simulink model "PID_PFL_3D_winds"  (R2022b)
settings: Solver=ode15s  StartTime=0.0  StopTime=0.8803  RelTol=1e-3
values from neighbouring files (symbols this model uses):
  theta1x_in = pinput(4 : 3 + n)    [Animation_3D.m]    (also in Constraint_3D_WCW.m = pinput(4 : 3+n); Cost_3D_WCW.m = pinput(4 : 3+n))
  theta1y_in = pinput(4 + n : 3 + 2*n)    [Animation_3D.m]    (also in Constraint_3D_WCW.m = pinput(4+n : 3+2*n); Cost_3D_WCW.m = pinput(4+n : 3+2*n))
  theta2_in = pinput(4 + 2*n : 3 + 3*n)    [Animation_3D.m]    (also in Constraint_3D_WCW.m = pinput(4+2*n : 3+3*n); Cost_3D_WCW.m = pinput(4+2*n : 3+3*n))
  timeVec = linspace(0, simTime, n)'    [Animation_3D.m]    (also in Main_3D_WCW.m = linspace(0, xmin(1), n)')
undefined symbols (not defined in the file or in its folder): sigbuilder_block, windSpeed
libraries: nesl_utility x6, sm_lib x4, slpidlib x3, simulink_extras x1
(part 1 of 2)
settings Model: Creator=Lenovo  LastModifiedBy=Stanley Mbewe
settings OptimizationCC: ReuseModelBlockBuffer=on

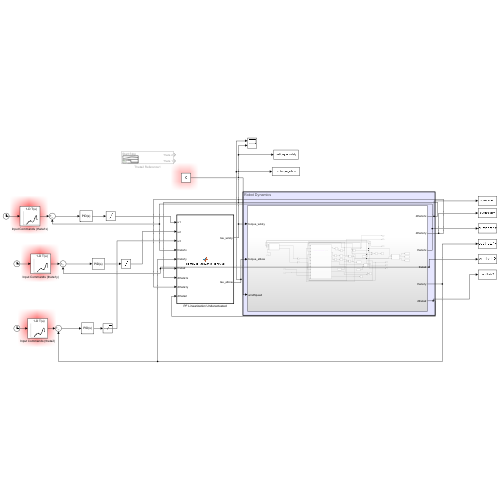
[thumbnail: Simulink's stored preview of the top-level diagram]
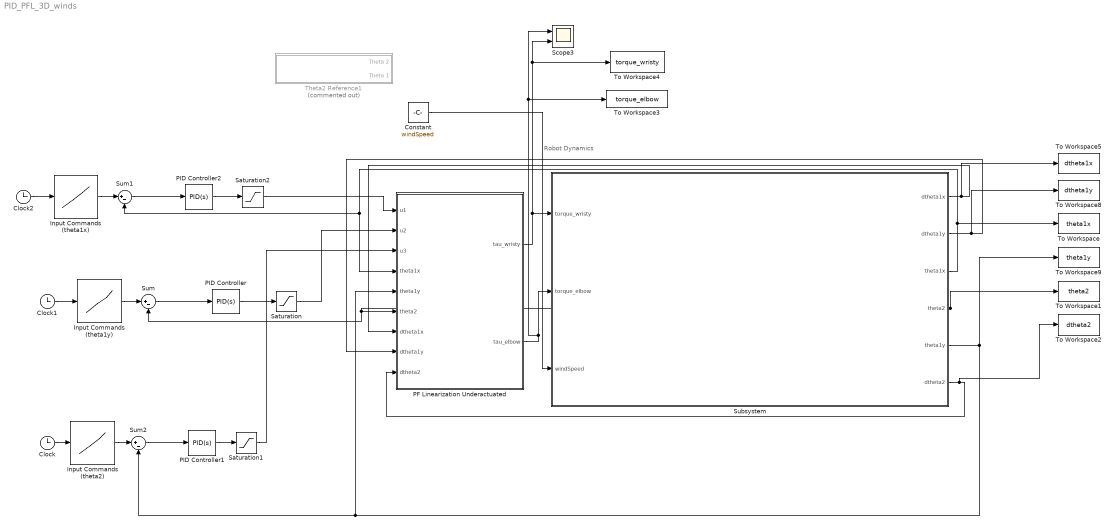
== system PID_PFL_3D_winds ==
  note: Robot Dynamics
  Clock : Clock
  Clock1 : Clock
  Clock2 : Clock
  Constant : Constant  Value=windSpeed
  Input Commands (theta1x) : Lookup_n-D  NumberOfTableDimensions=1  BreakpointsForDimension1=timeVec  Table=theta1x_in  InterpMethod=Cubic spline  InternalRulePriority=Speed  RndMeth=Simplest
  Input Commands (theta1y) : Lookup_n-D  NumberOfTableDimensions=1  BreakpointsForDimension1=timeVec  Table=theta1y_in  InterpMethod=Cubic spline  InternalRulePriority=Speed  RndMeth=Simplest
  Input Commands (theta2) : Lookup_n-D  NumberOfTableDimensions=1  LookupTableObject=theta1_in  BreakpointsForDimension1=timeVec  Table=theta2_in  InterpMethod=Cubic spline  InternalRulePriority=Speed  RndMeth=Simplest
  PF Linearization Underactuated : MATLAB Function  TreatAsAtomicUnit=on
  PID Controller : slpidlib/PID Controller  Controller=PID  Form=Parallel  TimeDomain=Continuous-time  UseExternalTs=off  SampleTime=-1  IntegratorMethod=Forward Euler  FilterMethod=Forward Euler  ControllerParametersSource=internal  P=149  I=10.1896438485082  UseKiTs=off  D=114  N=100  UseFilter=on  TunerSelectOption=Transfer Function Based (PID Tuner App)  InitialConditionSource=internal  InitialConditionForIntegrator=0  InitialConditionForFilter=0  DifferentiatorICPrevScaledInput=0  ExternalReset=none  TrackingMode=off  Kt=1  LimitOutput=off  SatLimitsSource=internal  UpperSaturationLimit=inf  LowerSaturationLimit=-inf  LinearizeAsGain=on  AntiWindupMode=none  Kb=1  LimitIntegrator=off  UpperIntegratorSaturationLimit=inf  LowerIntegratorSaturationLimit=-inf  POutMin=[]  POutMax=[]  IOutMin=[]  IOutMax=[]  DOutMin=[]  DOutMax=[]  NOutMin=[]  NOutMax=[]  SumOutMin=[]  SumOutMax=[]  SaturationOutMin=[]  SaturationOutMax=[]  PParamMin=[]  PParamMax=[]  IParamMin=[]  IParamMax=[]  DParamMin=[]  DParamMax=[]  NParamMin=[]  NParamMax=[]  KbParamMin=[]  KbParamMax=[]  KtParamMin=[]  KtParamMax=[]  KbOutMin=[]  KbOutMax=[]  KtOutMin=[]  KtOutMax=[]  IntegratorOutMin=[]  IntegratorOutMax=[]  FilterOutMin=[]  FilterOutMax=[]  SumI1OutMin=[]  SumI1OutMax=[]  SumI2OutMin=[]  SumI2OutMax=[]  SumI3OutMin=[]  SumI3OutMax=[]  SumI4OutMin=[]  SumI4OutMax=[]  SumDOutMin=[]  SumDOutMax=[]  DifferentiatorOutMin=[]  DifferentiatorOutMax=[]  FilterDiffOutCoefMin=[]  FilterDiffOutCoefMax=[]  ReciprocalOutMin=[]  ReciprocalOutMax=[]  SumDenOutMin=[]  SumDenOutMax=[]  SumNumOutMin=[]  SumNumOutMax=[]  DivideOutMin=[]  DivideOutMax=[]  UdiffTsProdOutMin=[]  UdiffTsProdOutMax=[]  NTsProdOutMin=[]  NTsProdOutMax=[]  UintegralTsProdOutMin=[]  UintegralTsProdOutMax=[]  UngainTsProdOutMin=[]  UngainTsProdOutMax=[]  ClampingZeroOutDataTypeStr=Inherit: Inherit via back propagation  ClampingZeroOutMin=[]  ClampingZeroOutMax=[]  FilterDenConstantOutDataTypeStr=Inherit: Inherit via back propagation  FilterDenConstantOutMin=[]  FilterDenConstantOutMax=[]  PCopyOutDataTypeStr=Inherit: Inherit via back propagation  PCopyOutMin=[]  PCopyOutMax=[]  NCopyOutDataTypeStr=Inherit: Inherit via back propagation  NCopyOutMin=[]  NCopyOutMax=[]  IntegratorContinuousStateAttributes=''  IntegratorStateMustResolveToSignalObject=off  IntegratorRTWStateStorageClass=Auto  FilterContinuousStateAttributes=''  FilterStateMustResolveToSignalObject=off  FilterRTWStateStorageClass=Auto  ParallelPVariant=InternalParameters  IdealPVariant=Disabled  IVariant=InternalParameters  DVariant=InternalParameters  IntegratorVariant=Continuous  SatVariant=Disabled  AWVariant=Passthrough  PCopyVariant=Disabled  TRVariant=Disabled  FdbkBlocksVariant=Forward  IdealPFdbkVariant=Disabled  SatFdbkVariant=Disabled  DerivativeFilterVariant=ContFilter  NVariant=InternalParameters  NCopyVariant=Disabled  FilterICVariant=InternalICsFilter  IntegratorICVariant=InternalICs  ExternalResetVariant=Disabled  TRSumVariant=Passthrough  SumFdbkVariant=Disabled  SumVariant=Sum_PID  TsampFilterVariant=InternalTs  TsampNgainVariant=Passthrough  TsampIntegralVariant=Passthrough  ExternalSaturationOutDataTypeStr=Inherit: Same as second input
  PID Controller1 : slpidlib/PID Controller  Controller=PID  Form=Parallel  TimeDomain=Continuous-time  UseExternalTs=off  SampleTime=-1  IntegratorMethod=Forward Euler  FilterMethod=Forward Euler  ControllerParametersSource=internal  P=149  I=10.1896438485082  UseKiTs=off  D=114  N=100  UseFilter=on  TunerSelectOption=Transfer Function Based (PID Tuner App)  InitialConditionSource=internal  InitialConditionForIntegrator=0  InitialConditionForFilter=0  DifferentiatorICPrevScaledInput=0  ExternalReset=none  TrackingMode=off  Kt=1  LimitOutput=off  SatLimitsSource=internal  UpperSaturationLimit=inf  LowerSaturationLimit=-inf  LinearizeAsGain=on  AntiWindupMode=none  Kb=1  LimitIntegrator=off  UpperIntegratorSaturationLimit=inf  LowerIntegratorSaturationLimit=-inf  POutMin=[]  POutMax=[]  IOutMin=[]  IOutMax=[]  DOutMin=[]  DOutMax=[]  NOutMin=[]  NOutMax=[]  SumOutMin=[]  SumOutMax=[]  SaturationOutMin=[]  SaturationOutMax=[]  PParamMin=[]  PParamMax=[]  IParamMin=[]  IParamMax=[]  DParamMin=[]  DParamMax=[]  NParamMin=[]  NParamMax=[]  KbParamMin=[]  KbParamMax=[]  KtParamMin=[]  KtParamMax=[]  KbOutMin=[]  KbOutMax=[]  KtOutMin=[]  KtOutMax=[]  IntegratorOutMin=[]  IntegratorOutMax=[]  FilterOutMin=[]  FilterOutMax=[]  SumI1OutMin=[]  SumI1OutMax=[]  SumI2OutMin=[]  SumI2OutMax=[]  SumI3OutMin=[]  SumI3OutMax=[]  SumI4OutMin=[]  SumI4OutMax=[]  SumDOutMin=[]  SumDOutMax=[]  DifferentiatorOutMin=[]  DifferentiatorOutMax=[]  FilterDiffOutCoefMin=[]  FilterDiffOutCoefMax=[]  ReciprocalOutMin=[]  ReciprocalOutMax=[]  SumDenOutMin=[]  SumDenOutMax=[]  SumNumOutMin=[]  SumNumOutMax=[]  DivideOutMin=[]  DivideOutMax=[]  UdiffTsProdOutMin=[]  UdiffTsProdOutMax=[]  NTsProdOutMin=[]  NTsProdOutMax=[]  UintegralTsProdOutMin=[]  UintegralTsProdOutMax=[]  UngainTsProdOutMin=[]  UngainTsProdOutMax=[]  ClampingZeroOutDataTypeStr=Inherit: Inherit via back propagation  ClampingZeroOutMin=[]  ClampingZeroOutMax=[]  FilterDenConstantOutDataTypeStr=Inherit: Inherit via back propagation  FilterDenConstantOutMin=[]  FilterDenConstantOutMax=[]  PCopyOutDataTypeStr=Inherit: Inherit via back propagation  PCopyOutMin=[]  PCopyOutMax=[]  NCopyOutDataTypeStr=Inherit: Inherit via back propagation  NCopyOutMin=[]  NCopyOutMax=[]  IntegratorContinuousStateAttributes=''  IntegratorStateMustResolveToSignalObject=off  IntegratorRTWStateStorageClass=Auto  FilterContinuousStateAttributes=''  FilterStateMustResolveToSignalObject=off  FilterRTWStateStorageClass=Auto  ParallelPVariant=InternalParameters  IdealPVariant=Disabled  IVariant=InternalParameters  DVariant=InternalParameters  IntegratorVariant=Continuous  SatVariant=Disabled  AWVariant=Passthrough  PCopyVariant=Disabled  TRVariant=Disabled  FdbkBlocksVariant=Forward  IdealPFdbkVariant=Disabled  SatFdbkVariant=Disabled  DerivativeFilterVariant=ContFilter  NVariant=InternalParameters  NCopyVariant=Disabled  FilterICVariant=InternalICsFilter  IntegratorICVariant=InternalICs  ExternalResetVariant=Disabled  TRSumVariant=Passthrough  SumFdbkVariant=Disabled  SumVariant=Sum_PID  TsampFilterVariant=InternalTs  TsampNgainVariant=Passthrough  TsampIntegralVariant=Passthrough  ExternalSaturationOutDataTypeStr=Inherit: Same as second input
  PID Controller2 : slpidlib/PID Controller  Controller=PID  Form=Parallel  TimeDomain=Continuous-time  UseExternalTs=off  SampleTime=-1  IntegratorMethod=Forward Euler  FilterMethod=Forward Euler  ControllerParametersSource=internal  P=149  I=10.1896438485082  UseKiTs=off  D=114  N=100  UseFilter=on  TunerSelectOption=Transfer Function Based (PID Tuner App)  InitialConditionSource=internal  InitialConditionForIntegrator=0  InitialConditionForFilter=0  DifferentiatorICPrevScaledInput=0  ExternalReset=none  TrackingMode=off  Kt=1  LimitOutput=off  SatLimitsSource=internal  UpperSaturationLimit=inf  LowerSaturationLimit=-inf  LinearizeAsGain=on  AntiWindupMode=none  Kb=1  LimitIntegrator=off  UpperIntegratorSaturationLimit=inf  LowerIntegratorSaturationLimit=-inf  POutMin=[]  POutMax=[]  IOutMin=[]  IOutMax=[]  DOutMin=[]  DOutMax=[]  NOutMin=[]  NOutMax=[]  SumOutMin=[]  SumOutMax=[]  SaturationOutMin=[]  SaturationOutMax=[]  PParamMin=[]  PParamMax=[]  IParamMin=[]  IParamMax=[]  DParamMin=[]  DParamMax=[]  NParamMin=[]  NParamMax=[]  KbParamMin=[]  KbParamMax=[]  KtParamMin=[]  KtParamMax=[]  KbOutMin=[]  KbOutMax=[]  KtOutMin=[]  KtOutMax=[]  IntegratorOutMin=[]  IntegratorOutMax=[]  FilterOutMin=[]  FilterOutMax=[]  SumI1OutMin=[]  SumI1OutMax=[]  SumI2OutMin=[]  SumI2OutMax=[]  SumI3OutMin=[]  SumI3OutMax=[]  SumI4OutMin=[]  SumI4OutMax=[]  SumDOutMin=[]  SumDOutMax=[]  DifferentiatorOutMin=[]  DifferentiatorOutMax=[]  FilterDiffOutCoefMin=[]  FilterDiffOutCoefMax=[]  ReciprocalOutMin=[]  ReciprocalOutMax=[]  SumDenOutMin=[]  SumDenOutMax=[]  SumNumOutMin=[]  SumNumOutMax=[]  DivideOutMin=[]  DivideOutMax=[]  UdiffTsProdOutMin=[]  UdiffTsProdOutMax=[]  NTsProdOutMin=[]  NTsProdOutMax=[]  UintegralTsProdOutMin=[]  UintegralTsProdOutMax=[]  UngainTsProdOutMin=[]  UngainTsProdOutMax=[]  ClampingZeroOutDataTypeStr=Inherit: Inherit via back propagation  ClampingZeroOutMin=[]  ClampingZeroOutMax=[]  FilterDenConstantOutDataTypeStr=Inherit: Inherit via back propagation  FilterDenConstantOutMin=[]  FilterDenConstantOutMax=[]  PCopyOutDataTypeStr=Inherit: Inherit via back propagation  PCopyOutMin=[]  PCopyOutMax=[]  NCopyOutDataTypeStr=Inherit: Inherit via back propagation  NCopyOutMin=[]  NCopyOutMax=[]  IntegratorContinuousStateAttributes=''  IntegratorStateMustResolveToSignalObject=off  IntegratorRTWStateStorageClass=Auto  FilterContinuousStateAttributes=''  FilterStateMustResolveToSignalObject=off  FilterRTWStateStorageClass=Auto  ParallelPVariant=InternalParameters  IdealPVariant=Disabled  IVariant=InternalParameters  DVariant=InternalParameters  IntegratorVariant=Continuous  SatVariant=Disabled  AWVariant=Passthrough  PCopyVariant=Disabled  TRVariant=Disabled  FdbkBlocksVariant=Forward  IdealPFdbkVariant=Disabled  SatFdbkVariant=Disabled  DerivativeFilterVariant=ContFilter  NVariant=InternalParameters  NCopyVariant=Disabled  FilterICVariant=InternalICsFilter  IntegratorICVariant=InternalICs  ExternalResetVariant=Disabled  TRSumVariant=Passthrough  SumFdbkVariant=Disabled  SumVariant=Sum_PID  TsampFilterVariant=InternalTs  TsampNgainVariant=Passthrough  TsampIntegralVariant=Passthrough  ExternalSaturationOutDataTypeStr=Inherit: Same as second input
  Saturation : Saturate  UpperLimit=10  LowerLimit=-10
  Saturation1 : Saturate  UpperLimit=50  LowerLimit=-50
  Saturation2 : Saturate  UpperLimit=10  LowerLimit=-10
  Scope3 : Scope  NumInputPorts=2
  Subsystem : Subsystem
  Sum : Sum  Inputs=|+-
  Sum1 : Sum  Inputs=|+-
  Sum2 : Sum  Inputs=|+-
  Theta2 Reference1 : Subsystem  Tag=STV Subsys  Commented=on  LoadFcn=sigbuilder_block('load');  StartFcn=sigbuilder_block('start');  StopFcn=sigbuilder_block('stop');  ClipboardFcn=sigbuilder_block('clipboard');  mask(Sigbuilder block){tuvar=[0:10]}
      mask help: Sigbuilder GUI
      mask init:
      | if ~strcmp(get_param(bdroot(gcbh),'SimulationStatus'),'stopped') tuvar = sigbuilder_block('maskInit'); end
      settings: CopyFcn=sigbuilder_block('copy');  DeleteFcn=sigbuilder_block('delete');  ModelCloseFcn=sigbuilder_block('modelClose');  PreSaveFcn=sigbuilder_block('preSave');  PauseFcn=sigbuilder_block('pause')  ContinueFcn=sigbuilder_block('continue')  NameChangeFcn=sigbuilder_block('namechange');  OpenFcn=sigbuilder_block('open',[200.4 71.4 762 360.6 ]);  CloseFcn=sigbuilder_block('close');
      mask Display: plot(0, 0, 100, 100,[2, 2, 32, 32, 2], [68, 8, 8, 68, 68],[32, 2], [38, 38], [32, 19, 2],[53, 60, 44], [32, 17, 17, 2],[16, 16, 31, 31]);txt = getActiveGroup(gcbh);text(2, 100, txt,'verticalAlignment', 'top');
  To Workspace : ToWorkspace  VariableName=theta1x  SampleTime=0.01
  To Workspace1 : ToWorkspace  VariableName=theta2  SampleTime=0.01
  To Workspace2 : ToWorkspace  VariableName=dtheta2  SampleTime=0.01
  To Workspace3 : ToWorkspace  VariableName=torque_elbow  SampleTime=0.01
  To Workspace4 : ToWorkspace  VariableName=torque_wristy  SampleTime=0.01
  To Workspace5 : ToWorkspace  VariableName=dtheta1x  SampleTime=0.01
  To Workspace8 : ToWorkspace  VariableName=dtheta1y  SampleTime=0.01
  To Workspace9 : ToWorkspace  VariableName=theta1y  SampleTime=0.01
  wires:
  Sum/1 -> PID Controller/1
  Sum2/1 -> PID Controller1/1
  PID Controller/1 -> Saturation/1
  PID Controller1/1 -> Saturation1/1
  Clock/1 -> Input Commands (theta2)/1
  Clock1/1 -> Input Commands (theta1y)/1
  PF Linearization Underactuated/1(tau_wristy) -> To Workspace4/1, Scope3/2, Subsystem/1(torque_wristy)
  PF Linearization Underactuated/2(tau_elbow) -> Scope3/1, To Workspace3/1, Subsystem/2(torque_elbow)
  Subsystem/4(theta2) -> To Workspace1/1, PF Linearization Underactuated/6(theta2), Sum/2
  Subsystem/5(theta1y) -> PF Linearization Underactuated/5(theta1y), Sum2/2, To Workspace9/1
  Subsystem/3(theta1x) -> To Workspace/1, Sum1/2, PF Linearization Underactuated/4(theta1x)
  Subsystem/1(dtheta1x) -> To Workspace5/1, PF Linearization Underactuated/7(dtheta1x)
  Subsystem/2(dtheta1y) -> To Workspace8/1, PF Linearization Underactuated/8(dtheta1y)
  Subsystem/6(dtheta2) -> To Workspace2/1, PF Linearization Underactuated/9(dtheta2)
  Input Commands (theta2)/1 -> Sum2/1
  Input Commands (theta1y)/1 -> Sum/1
  Input Commands (theta1x)/1 -> Sum1/1
  Clock2/1 -> Input Commands (theta1x)/1
  PID Controller2/1 -> Saturation2/1
  Sum1/1 -> PID Controller2/1
  Saturation2/1 -> PF Linearization Underactuated/1(u1)
  Saturation/1 -> PF Linearization Underactuated/2(u2)
  Saturation1/1 -> PF Linearization Underactuated/3(u3)
  Constant/1 -> Subsystem/3(windSpeed)

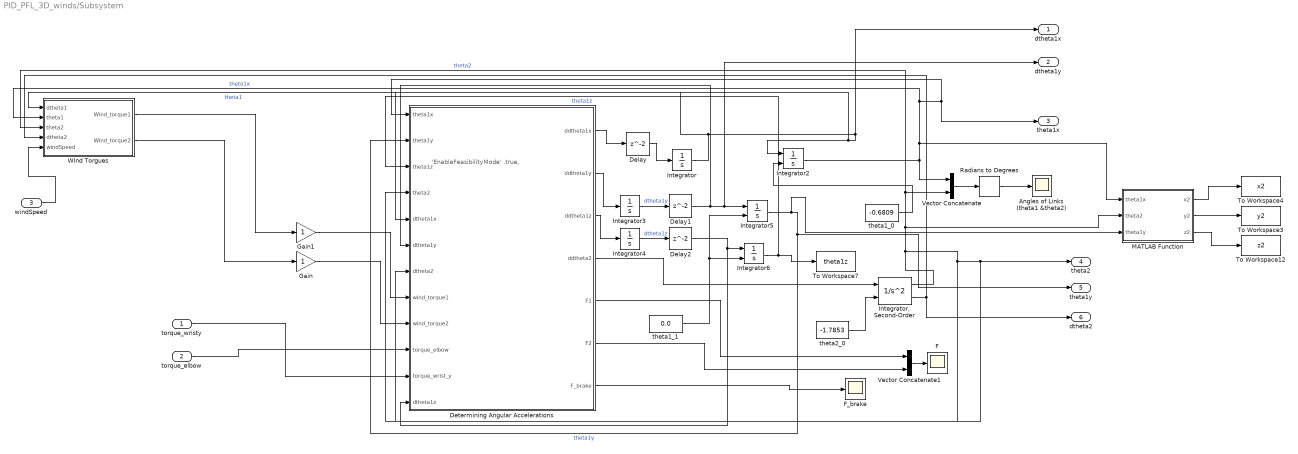
== system PID_PFL_3D_winds/Subsystem ==
  note: 'EnableFeasibilityMode' ,true,
  torque_wristy : Inport
  torque_elbow : Inport  Port=2
  windSpeed : Inport  Port=3
  Angles of Links (theta1 &theta2) : Scope
  Delay : Delay
  Delay1 : Delay
  Delay2 : Delay
  "Determining Angular Accelerations " : MATLAB Function  TreatAsAtomicUnit=on
  F : Scope
  F_brake : Scope
  Gain : Gain
  Gain1 : Gain
  Integrator : Integrator
  "Integrator, Second-Order" : SecondOrderIntegrator  ICSourceX=external  LimitX=on  UpperLimitX=160/(180/pi)  LowerLimitX=-160/(180/pi)  LimitDXDT=on  ReinitDXDTwhenXreachesSaturation=on
  Integrator2 : Integrator  InitialConditionSource=external
  Integrator3 : Integrator
  Integrator4 : Integrator
  Integrator5 : Integrator  InitialConditionSource=external
  Integrator6 : Integrator  InitialConditionSource=external
  MATLAB Function : MATLAB Function  TreatAsAtomicUnit=on
  Radians to Degrees : simulink_extras/Transformations/Radians to Degrees
  To Workspace12 : ToWorkspace  VariableName=z2  SampleTime=0.01
  To Workspace3 : ToWorkspace  VariableName=y2  SampleTime=0.01
  To Workspace4 : ToWorkspace  VariableName=x2  SampleTime=0.01
  To Workspace7 : ToWorkspace  VariableName=theta1z  SampleTime=0.01
  Vector Concatenate : Concatenate
  Vector Concatenate1 : Concatenate
  WInd Torgues : Subsystem
  theta1_0 : Constant  Value=-0.6809
  theta1_1 : Constant  Value=0.0
  theta2_0 : Constant  Value=-1.7853
  dtheta1x : Outport
  dtheta1y : Outport  Port=2
  theta1x : Outport  Port=3
  theta2 : Outport  Port=4
  theta1y : Outport  Port=5
  dtheta2 : Outport  Port=6
  wires:
  WInd Torgues/2(Wind_torque2) -> Gain/1
  Vector Concatenate/1 -> Radians to Degrees/1
  MATLAB Function/3(z2) -> To Workspace12/1
  Integrator5/1 -> MATLAB Function/3(theta1y), theta1y/1, "Determining Angular Accelerations "/2(theta1y)  "theta1y"
  "Integrator, Second-Order"/1 -> MATLAB Function/2(theta2), WInd Torgues/3(theta2), Vector Concatenate/2, "Determining Angular Accelerations "/4(theta2), theta2/1, "Determining Angular Accelerations "/7(dtheta2)  "theta2"
  Integrator6/1 -> To Workspace7/1, "Determining Angular Accelerations "/3(theta1z)  "theta1z"
  "Determining Angular Accelerations "/6(F2) -> Vector Concatenate1/2
  "Determining Angular Accelerations "/4(ddtheta2) -> "Integrator, Second-Order"/1
  "Integrator, Second-Order"/2 -> dtheta2/1, WInd Torgues/4(dtheta2)
  Integrator2/1 -> MATLAB Function/1(theta1x), theta1x/1, "Determining Angular Accelerations "/1(theta1x), WInd Torgues/2(theta1), Vector Concatenate/1  "theta1x"
  "Determining Angular Accelerations "/7(F_brake) -> F_brake/1
  Delay2/1 -> "Determining Angular Accelerations "/12(dtheta1z), Integrator6/1
  "Determining Angular Accelerations "/5(F1) -> Vector Concatenate1/1
  Integrator4/1 -> Delay2/1  "dtheta1z"
  Integrator/1 -> dtheta1x/1, Integrator2/1, WInd Torgues/1(dtheta1), "Determining Angular Accelerations "/5(dtheta1x)  "theta1"
  theta1_1/1 -> Integrator5/2, Integrator6/2
  Radians to Degrees/1 -> Angles of Links (theta1 &theta2)/1
  Gain1/1 -> "Determining Angular Accelerations "/8(wind_torque1)
  WInd Torgues/1(Wind_torque1) -> Gain1/1
  MATLAB Function/2(y2) -> To Workspace3/1
  MATLAB Function/1(x2) -> To Workspace4/1
  Vector Concatenate1/1 -> F/1
  Delay1/1 -> "Determining Angular Accelerations "/6(dtheta1y), dtheta1y/1, Integrator5/1
  theta1_0/1 -> Integrator2/2
  Integrator3/1 -> Delay1/1  "dtheta1y"
  Delay/1 -> Integrator/1
  "Determining Angular Accelerations "/3(ddtheta1z) -> Integrator4/1
  "Determining Angular Accelerations "/1(ddtheta1x) -> Delay/1
  "Determining Angular Accelerations "/2(ddtheta1y) -> Integrator3/1
  theta2_0/1 -> "Integrator, Second-Order"/2
  Gain/1 -> "Determining Angular Accelerations "/9(wind_torque2)
  torque_wristy/1 -> "Determining Angular Accelerations "/11(torque_wrist_y)
  torque_elbow/1 -> "Determining Angular Accelerations "/10(torque_elbow)
  windSpeed/1 -> WInd Torgues/5(windSpeed)

== system PID_PFL_3D_winds/Theta2 Reference1 ==
  Demux : Demux  Tag=STV Demux  Outputs=2
      settings: DisplayOption=none
  FromWs : FromWorkspace  Tag=STV FromWs  VariableName=tuvar
  Theta 2 : Outport  Tag=STV Outport
  Theta 1 : Outport  Tag=STV Outport  Port=2
  wires:
  Demux/2 -> Theta 1/1
  Demux/1 -> Theta 2/1
  FromWs/1 -> Demux/1

== system PID_PFL_3D_winds/Subsystem/WInd Torgues ==
  dtheta1 : Inport
  theta1 : Inport  Port=2
  theta2 : Inport  Port=3
  dtheta2 : Inport  Port=4
  windSpeed : Inport  Port=5
  Unsteady Wind Velocities : MATLAB Function  TreatAsAtomicUnit=on
  Wind loadind : Subsystem
  Wind_torque1 : Outport
  Wind_torque2 : Outport  Port=2
  wires:
  Unsteady Wind Velocities/2(U_R2) -> Wind loadind/6(WindSpeed2)
  Wind loadind/2(Wind_torque2) -> Wind_torque2/1
  Unsteady Wind Velocities/1(U_R1) -> Wind loadind/5(WindSpeed1)
  Wind loadind/1(Wind_torque1) -> Wind_torque1/1
  theta1/1 -> Wind loadind/1(theta1)
  dtheta1/1 -> Wind loadind/3(dtheta1)
  theta2/1 -> Wind loadind/2(theta2)
  dtheta2/1 -> Wind loadind/4(dtheta2)
  windSpeed/1 -> Unsteady Wind Velocities/1(windSpeed)

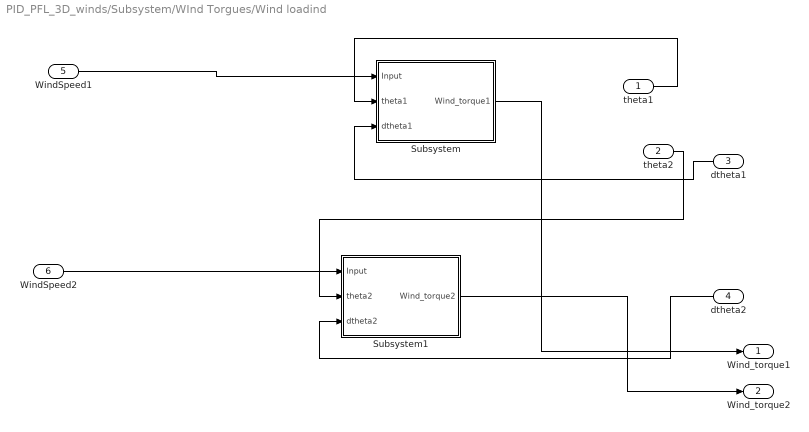
== system PID_PFL_3D_winds/Subsystem/WInd Torgues/Wind loadind ==
  theta1 : Inport
  theta2 : Inport  Port=2
  dtheta1 : Inport  Port=3
  dtheta2 : Inport  Port=4
  WindSpeed1 : Inport  Port=5
  WindSpeed2 : Inport  Port=6
  Subsystem : Subsystem  VariantControl=Choice
  Subsystem1 : Subsystem  VariantControl=Choice
  Wind_torque1 : Outport
  Wind_torque2 : Outport  Port=2
  wires:
  dtheta2/1 -> Subsystem1/3(dtheta2)
  dtheta1/1 -> Subsystem/3(dtheta1)
  theta1/1 -> Subsystem/2(theta1)
  Subsystem1/1(Wind_torque2) -> Wind_torque2/1
  theta2/1 -> Subsystem1/2(theta2)
  Subsystem/1(Wind_torque1) -> Wind_torque1/1
  WindSpeed1/1 -> Subsystem/1(Input)
  WindSpeed2/1 -> Subsystem1/1(Input)

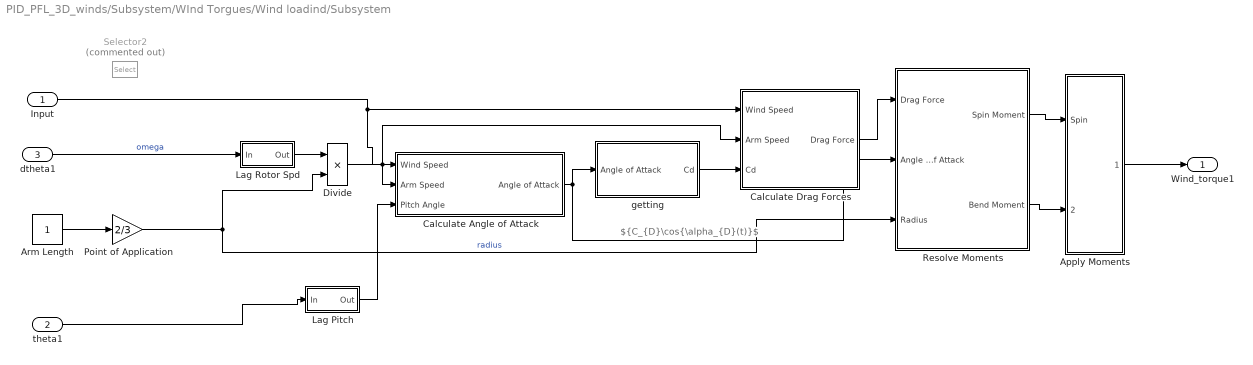
== system PID_PFL_3D_winds/Subsystem/WInd Torgues/Wind loadind/Subsystem ==
  note: ${C_{D}\cos{\alpha_{D}(t)}$
  Input : Inport
  theta1 : Inport  Port=2
  dtheta1 : Inport  Port=3
  Apply Moments : Subsystem
  Arm Length : Constant
  Calculate Drag Forces : Subsystem
  Calculate Angle of Attack : Subsystem
  Divide : Product  Inputs=**
  Lag Pitch : Subsystem  mask(First-order lag supporting vector signals){b=0.01, x_initial=0}
      mask prompts: b "Filter time constant"; x_initial "Initial output"
      mask help: Models a lag of the form 1/(b*s+1) where s is the Laplace operator.
  Lag Rotor Spd : Subsystem  mask(First-order lag supporting vector signals){b=0.01, x_initial=0}
      mask prompts: b "Filter time constant"; x_initial "Initial output"
      mask help: Models a lag of the form 1/(b*s+1) where s is the Laplace operator.
  Point of Application : Gain  Gain=2/3
  Resolve Moments : Subsystem
  Selector2 : Selector  Commented=on  InputPortWidth=2  IndexOptions=Index vector (dialog)  Indices=[1]  OutputSizes=1
  "getting " : Subsystem
  Wind_torque1 : Outport
  wires:
  Divide/1 -> Calculate Drag Forces/2(Arm Speed), Calculate Angle of Attack/2(Arm Speed)
  theta1/1 -> Lag Pitch/1(In)
  Arm Length/1 -> Point of Application/1
  Lag Pitch/1(Out) -> Calculate Angle of Attack/3(Pitch Angle)
  Point of Application/1 -> Divide/2, Resolve Moments/3(Radius)  "radius"
  Calculate Drag Forces/1(Drag Force) -> Resolve Moments/1(Drag Force)
  Resolve Moments/1(Spin Moment) -> Apply Moments/1(Spin)
  Resolve Moments/2(Bend Moment) -> Apply Moments/2(Bend)
  Calculate Angle of Attack/1(Angle of Attack) -> "getting "/1(Angle of Attack), Resolve Moments/2(Angle of Attack)
  Lag Rotor Spd/1(Out) -> Divide/1
  "getting "/1(Cd) -> Calculate Drag Forces/3(Cd)
  dtheta1/1 -> Lag Rotor Spd/1(In)  "omega"
  Apply Moments/1(Torque) -> Wind_torque1/1
  Input/1 -> Calculate Drag Forces/1(Wind Speed), Calculate Angle of Attack/1(Wind Speed)

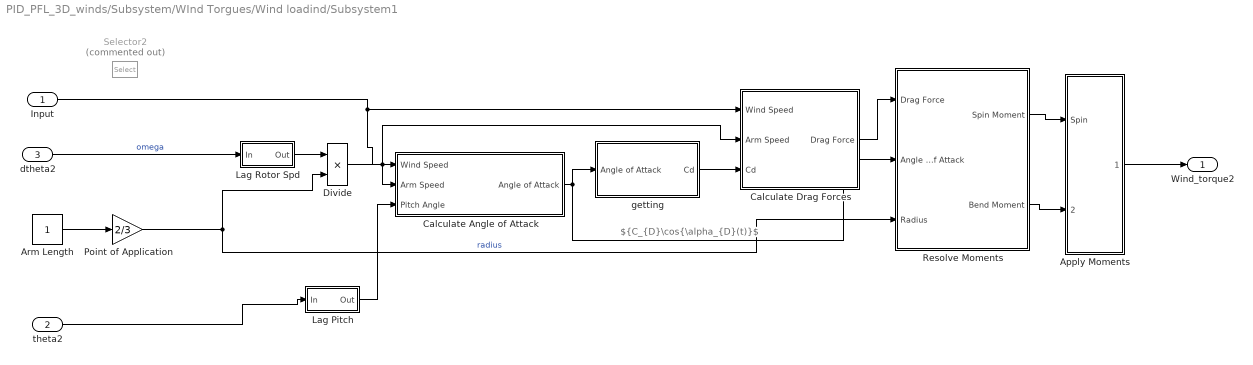
== system PID_PFL_3D_winds/Subsystem/WInd Torgues/Wind loadind/Subsystem1 ==
  note: ${C_{D}\cos{\alpha_{D}(t)}$
  Input : Inport
  theta2 : Inport  Port=2
  dtheta2 : Inport  Port=3
  Apply Moments : Subsystem
  Arm Length : Constant
  Calculate Drag Forces : Subsystem
  Calculate Angle of Attack : Subsystem
  Divide : Product  Inputs=**
  Lag Pitch : Subsystem  mask(First-order lag supporting vector signals){b=0.01, x_initial=0}
      mask prompts: b "Filter time constant"; x_initial "Initial output"
      mask help: Models a lag of the form 1/(b*s+1) where s is the Laplace operator.
  Lag Rotor Spd : Subsystem  mask(First-order lag supporting vector signals){b=0.01, x_initial=0}
      mask prompts: b "Filter time constant"; x_initial "Initial output"
      mask help: Models a lag of the form 1/(b*s+1) where s is the Laplace operator.
  Point of Application : Gain  Gain=2/3
  Resolve Moments : Subsystem
  Selector2 : Selector  Commented=on  InputPortWidth=2  IndexOptions=Index vector (dialog)  Indices=[1]  OutputSizes=1
  "getting " : Subsystem
  Wind_torque2 : Outport
  wires:
  Input/1 -> Calculate Angle of Attack/1(Wind Speed), Calculate Drag Forces/1(Wind Speed)
  Apply Moments/1(Torque) -> Wind_torque2/1
  dtheta2/1 -> Lag Rotor Spd/1(In)  "omega"
  "getting "/1(Cd) -> Calculate Drag Forces/3(Cd)
  Lag Rotor Spd/1(Out) -> Divide/1
  Calculate Angle of Attack/1(Angle of Attack) -> Resolve Moments/2(Angle of Attack), "getting "/1(Angle of Attack)
  Resolve Moments/2(Bend Moment) -> Apply Moments/2(Bend)
  Resolve Moments/1(Spin Moment) -> Apply Moments/1(Spin)
  Calculate Drag Forces/1(Drag Force) -> Resolve Moments/1(Drag Force)
  Point of Application/1 -> Resolve Moments/3(Radius), Divide/2  "radius"
  Lag Pitch/1(Out) -> Calculate Angle of Attack/3(Pitch Angle)
  Arm Length/1 -> Point of Application/1
  theta2/1 -> Lag Pitch/1(In)
  Divide/1 -> Calculate Angle of Attack/2(Arm Speed), Calculate Drag Forces/2(Arm Speed)

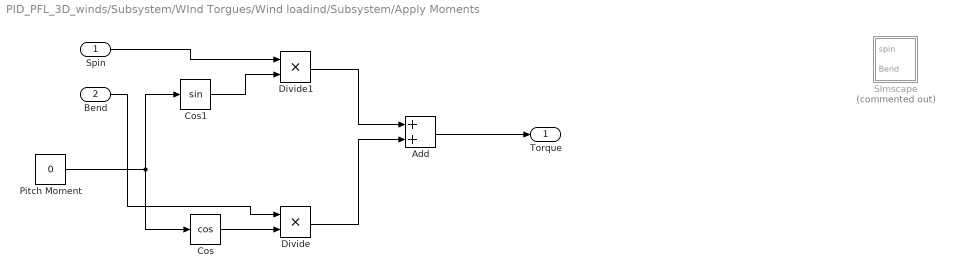
== system PID_PFL_3D_winds/Subsystem/WInd Torgues/Wind loadind/Subsystem/Apply Moments ==
  Spin : Inport
  Bend : Inport  Port=2
  Add : Sum
  Cos : Trigonometry  Operator=cos
  Cos1 : Trigonometry
  Divide : Product  Inputs=**
  Divide1 : Product  Inputs=**
  Pitch Moment : Constant  Value=0
  SImscape : Subsystem  Commented=on
  Torque : Outport
  wires:
  Pitch Moment/1 -> Cos1/1, Cos/1
  Spin/1 -> Divide1/1
  Cos1/1 -> Divide1/2
  Bend/1 -> Divide/1
  Cos/1 -> Divide/2
  Divide1/1 -> Add/1
  Divide/1 -> Add/2
  Add/1 -> Torque/1

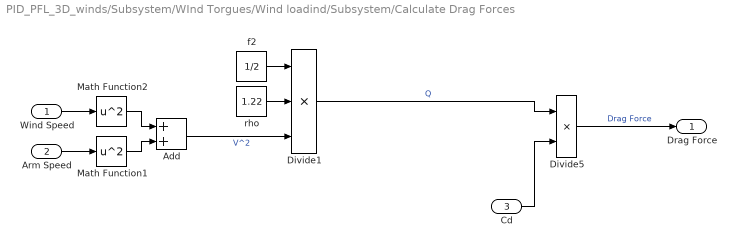
== system PID_PFL_3D_winds/Subsystem/WInd Torgues/Wind loadind/Subsystem/Calculate Drag Forces ==
  Wind Speed : Inport
  Arm Speed : Inport  Port=2
  Cd : Inport  Port=3
  Add : Sum
  Divide1 : Product  Inputs=***
  Divide5 : Product  Inputs=**
  Math Function1 : Math  Operator=square  SignedPower=on
  Math Function2 : Math  Operator=square  SignedPower=on
  f2 : Constant  Value=1/2
  rho : Constant  Value=1.22
  Drag Force : Outport  VectorParamsAs1DForOutWhenUnconnected=off
  wires:
  Cd/1 -> Divide5/2
  Divide5/1 -> Drag Force/1  "Drag Force"
  Arm Speed/1 -> Math Function1/1
  Wind Speed/1 -> Math Function2/1
  Divide1/1 -> Divide5/1  "Q"
  f2/1 -> Divide1/1
  rho/1 -> Divide1/2
  Add/1 -> Divide1/3  "V^2"
  Math Function1/1 -> Add/2
  Math Function2/1 -> Add/1

== system PID_PFL_3D_winds/Subsystem/WInd Torgues/Wind loadind/Subsystem/Calculate Angle of Attack ==
  Wind Speed : Inport
  Arm Speed : Inport  Port=2
  Pitch Angle : Inport  Port=3
  Subtract : Sum  Inputs=+-
  Trigonometric Function : Trigonometry  Operator=atan2
  Angle of Attack : Outport  VectorParamsAs1DForOutWhenUnconnected=off
  wires:
  Pitch Angle/1 -> Subtract/2  "theta"
  Subtract/1 -> Angle of Attack/1  "alpha"
  Arm Speed/1 -> Trigonometric Function/2
  Wind Speed/1 -> Trigonometric Function/1
  Trigonometric Function/1 -> Subtract/1

== system PID_PFL_3D_winds/Subsystem/WInd Torgues/Wind loadind/Subsystem/Lag Pitch ==
  In : Inport
  Gain : Gain  Gain=100
  Integrator : Integrator  InitialCondition=x_initial
  Sum : Sum  Inputs=|+-  InputSameDT=on  SaturateOnIntegerOverflow=on  OutDataTypeStr=Inherit: Same as first input
  Out : Outport  VectorParamsAs1DForOutWhenUnconnected=off
  wires:
  Gain/1 -> Out/1, Sum/2
  Integrator/1 -> Gain/1
  In/1 -> Sum/1
  Sum/1 -> Integrator/1

== system PID_PFL_3D_winds/Subsystem/WInd Torgues/Wind loadind/Subsystem/Lag Rotor Spd ==
  In : Inport
  Gain : Gain  Gain=100
  Integrator : Integrator  InitialCondition=x_initial
  Sum : Sum  Inputs=|+-  InputSameDT=on  SaturateOnIntegerOverflow=on  OutDataTypeStr=Inherit: Same as first input
  Out : Outport  VectorParamsAs1DForOutWhenUnconnected=off
  wires:
  Sum/1 -> Integrator/1
  In/1 -> Sum/1
  Integrator/1 -> Gain/1
  Gain/1 -> Sum/2, Out/1

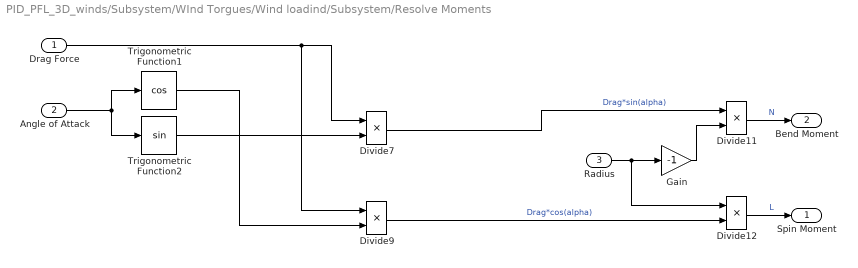
== system PID_PFL_3D_winds/Subsystem/WInd Torgues/Wind loadind/Subsystem/Resolve Moments ==
  Drag Force : Inport
  Angle of Attack : Inport  Port=2
  Radius : Inport  Port=3
  Divide{7,9,11..12} (4 alike) : Product  Inputs=**
  Gain : Gain  Gain=-1
  Trigonometric Function1 : Trigonometry  Operator=cos
  Trigonometric Function2 : Trigonometry
  Spin Moment : Outport  VectorParamsAs1DForOutWhenUnconnected=off
  Bend Moment : Outport  Port=2  VectorParamsAs1DForOutWhenUnconnected=off
  wires:
  Divide12/1 -> Spin Moment/1  "L"
  Divide11/1 -> Bend Moment/1  "N"
  Radius/1 -> Divide12/1, Gain/1
  Angle of Attack/1 -> Trigonometric Function2/1, Trigonometric Function1/1
  Gain/1 -> Divide11/2
  Divide9/1 -> Divide12/2  "Drag*cos(alpha)"
  Divide7/1 -> Divide11/1  "Drag*sin(alpha)"
  Trigonometric Function2/1 -> Divide7/2
  Trigonometric Function1/1 -> Divide9/2
  Drag Force/1 -> Divide9/1, Divide7/1

== system PID_PFL_3D_winds/Subsystem/WInd Torgues/Wind loadind/Subsystem/getting  ==
  Angle of Attack : Inport
  Cos : Trigonometry  Operator=cos
  Divide : Product  Inputs=**
  f1 : Constant  Value=0.82/2
  Cd : Outport  VectorParamsAs1DForOutWhenUnconnected=off
  wires:
  Divide/1 -> Cd/1  "CdCos(alpha)"
  f1/1 -> Divide/2
  Angle of Attack/1 -> Cos/1
  Cos/1 -> Divide/1

== system PID_PFL_3D_winds/Subsystem/WInd Torgues/Wind loadind/Subsystem1/Apply Moments ==
  Spin : Inport
  Bend : Inport  Port=2
  Add : Sum
  Cos : Trigonometry  Operator=cos
  Cos1 : Trigonometry
  Divide : Product  Inputs=**
  Divide1 : Product  Inputs=**
  Pitch Moment : Constant  Value=0
  SImscape : Subsystem  Commented=on
  Torque : Outport
  wires:
  Add/1 -> Torque/1
  Divide/1 -> Add/2
  Divide1/1 -> Add/1
  Cos/1 -> Divide/2
  Bend/1 -> Divide/1
  Cos1/1 -> Divide1/2
  Spin/1 -> Divide1/1
  Pitch Moment/1 -> Cos/1, Cos1/1

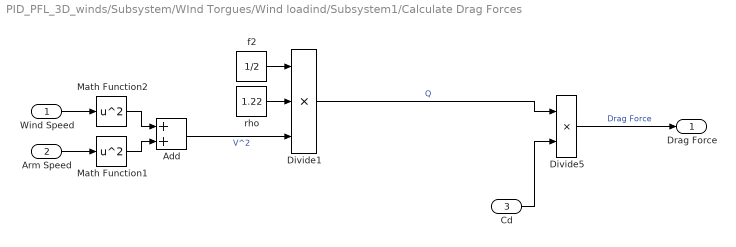
== system PID_PFL_3D_winds/Subsystem/WInd Torgues/Wind loadind/Subsystem1/Calculate Drag Forces ==
  Wind Speed : Inport
  Arm Speed : Inport  Port=2
  Cd : Inport  Port=3
  Add : Sum
  Divide1 : Product  Inputs=***
  Divide5 : Product  Inputs=**
  Math Function1 : Math  Operator=square  SignedPower=on
  Math Function2 : Math  Operator=square  SignedPower=on
  f2 : Constant  Value=1/2
  rho : Constant  Value=1.22
  Drag Force : Outport  VectorParamsAs1DForOutWhenUnconnected=off
  wires:
  Math Function2/1 -> Add/1
  Math Function1/1 -> Add/2
  Add/1 -> Divide1/3  "V^2"
  rho/1 -> Divide1/2
  f2/1 -> Divide1/1
  Divide1/1 -> Divide5/1  "Q"
  Wind Speed/1 -> Math Function2/1
  Arm Speed/1 -> Math Function1/1
  Divide5/1 -> Drag Force/1  "Drag Force"
  Cd/1 -> Divide5/2

== system PID_PFL_3D_winds/Subsystem/WInd Torgues/Wind loadind/Subsystem1/Calculate Angle of Attack ==
  Wind Speed : Inport
  Arm Speed : Inport  Port=2
  Pitch Angle : Inport  Port=3
  Subtract : Sum  Inputs=+-
  Trigonometric Function : Trigonometry  Operator=atan2
  Angle of Attack : Outport  VectorParamsAs1DForOutWhenUnconnected=off
  wires:
  Trigonometric Function/1 -> Subtract/1
  Wind Speed/1 -> Trigonometric Function/1
  Arm Speed/1 -> Trigonometric Function/2
  Subtract/1 -> Angle of Attack/1  "alpha"
  Pitch Angle/1 -> Subtract/2  "theta"

== system PID_PFL_3D_winds/Subsystem/WInd Torgues/Wind loadind/Subsystem1/Lag Pitch ==
  In : Inport
  Gain : Gain  Gain=100
  Integrator : Integrator  InitialCondition=x_initial
  Sum : Sum  Inputs=|+-  InputSameDT=on  SaturateOnIntegerOverflow=on  OutDataTypeStr=Inherit: Same as first input
  Out : Outport  VectorParamsAs1DForOutWhenUnconnected=off
  wires:
  Sum/1 -> Integrator/1
  In/1 -> Sum/1
  Integrator/1 -> Gain/1
  Gain/1 -> Sum/2, Out/1

== system PID_PFL_3D_winds/Subsystem/WInd Torgues/Wind loadind/Subsystem1/Lag Rotor Spd ==
  In : Inport
  Gain : Gain  Gain=100
  Integrator : Integrator  InitialCondition=x_initial
  Sum : Sum  Inputs=|+-  InputSameDT=on  SaturateOnIntegerOverflow=on  OutDataTypeStr=Inherit: Same as first input
  Out : Outport  VectorParamsAs1DForOutWhenUnconnected=off
  wires:
  Gain/1 -> Out/1, Sum/2
  Integrator/1 -> Gain/1
  In/1 -> Sum/1
  Sum/1 -> Integrator/1

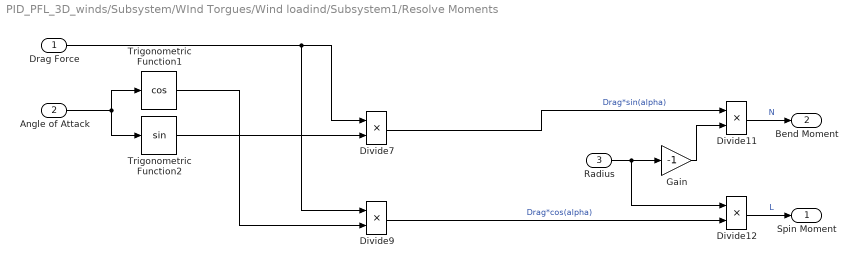
== system PID_PFL_3D_winds/Subsystem/WInd Torgues/Wind loadind/Subsystem1/Resolve Moments ==
  Drag Force : Inport
  Angle of Attack : Inport  Port=2
  Radius : Inport  Port=3
  Divide{7,9,11..12} (4 alike) : Product  Inputs=**
  Gain : Gain  Gain=-1
  Trigonometric Function1 : Trigonometry  Operator=cos
  Trigonometric Function2 : Trigonometry
  Spin Moment : Outport  VectorParamsAs1DForOutWhenUnconnected=off
  Bend Moment : Outport  Port=2  VectorParamsAs1DForOutWhenUnconnected=off
  wires:
  Drag Force/1 -> Divide7/1, Divide9/1
  Trigonometric Function1/1 -> Divide9/2
  Trigonometric Function2/1 -> Divide7/2
  Divide7/1 -> Divide11/1  "Drag*sin(alpha)"
  Divide9/1 -> Divide12/2  "Drag*cos(alpha)"
  Gain/1 -> Divide11/2
  Angle of Attack/1 -> Trigonometric Function1/1, Trigonometric Function2/1
  Radius/1 -> Gain/1, Divide12/1
  Divide11/1 -> Bend Moment/1  "N"
  Divide12/1 -> Spin Moment/1  "L"

== system PID_PFL_3D_winds/Subsystem/WInd Torgues/Wind loadind/Subsystem1/getting  ==
  Angle of Attack : Inport
  Cos : Trigonometry  Operator=cos
  Divide : Product  Inputs=**
  f1 : Constant  Value=0.82/2
  Cd : Outport  VectorParamsAs1DForOutWhenUnconnected=off
  wires:
  Cos/1 -> Divide/1
  Angle of Attack/1 -> Cos/1
  f1/1 -> Divide/2
  Divide/1 -> Cd/1  "CdCos(alpha)"

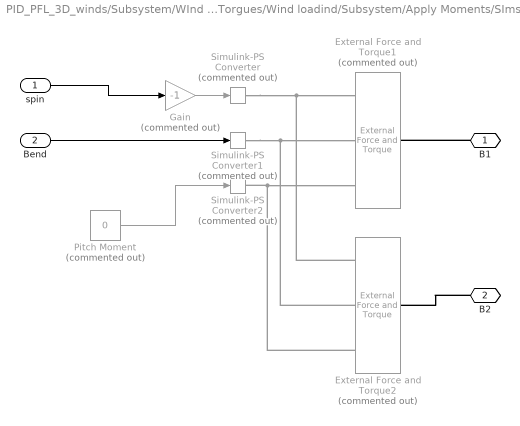
== system PID_PFL_3D_winds/Subsystem/WInd Torgues/Wind loadind/Subsystem/Apply Moments/SImscape ==
  spin : Inport
  Bend : Inport  Port=2
  External Force and Torque1 : sm_lib/Forces and Torques/External Force and Torque  Commented=on  ForceResolutionFrame=AttachedFrame  EnableForceX=off  EnableForceY=off  EnableForceZ=off  EnableForce=off  TorqueResolutionFrame=AttachedFrame  EnableTorqueX=on  EnableTorqueY=on  EnableTorqueZ=on  EnableTorque=off
  External Force and Torque2 : sm_lib/Forces and Torques/External Force and Torque  Commented=on  ForceResolutionFrame=AttachedFrame  EnableForceX=off  EnableForceY=off  EnableForceZ=off  EnableForce=off  TorqueResolutionFrame=AttachedFrame  EnableTorqueX=on  EnableTorqueY=on  EnableTorqueZ=on  EnableTorque=off
  Gain : Gain  Commented=on  Gain=-1
  Pitch Moment : Constant  Commented=on  Value=0
  Simulink-PS Converter : nesl_utility/Simulink-PS Converter  Commented=on  PhysicalDomain=network_engine_domain  SubClassName=ps_input  LeftPortType=input  RightPortType=output  PseudoPeriodic=off  Frequencies=[]  NoiseDistribution=none  NoiseParameters=[]  Unit=1  AffineConversion=off  FilteringAndDerivatives=zero  SimscapeFilterOrder=1  InputFilterTimeConstant=0.005  UdotUserProvided=[]
  Simulink-PS Converter1 : nesl_utility/Simulink-PS Converter  Commented=on  PhysicalDomain=network_engine_domain  SubClassName=ps_input  LeftPortType=input  RightPortType=output  PseudoPeriodic=off  Frequencies=[]  NoiseDistribution=none  NoiseParameters=[]  Unit=1  AffineConversion=off  FilteringAndDerivatives=zero  SimscapeFilterOrder=1  InputFilterTimeConstant=0.005  UdotUserProvided=[]
  Simulink-PS Converter2 : nesl_utility/Simulink-PS Converter  Commented=on  PhysicalDomain=network_engine_domain  SubClassName=ps_input  LeftPortType=input  RightPortType=output  PseudoPeriodic=off  Frequencies=[]  NoiseDistribution=none  NoiseParameters=[]  Unit=1  AffineConversion=off  FilteringAndDerivatives=zero  SimscapeFilterOrder=1  InputFilterTimeConstant=0.005  UdotUserProvided=[]
  B1 : PMIOPort  Side=Right
  B2 : PMIOPort  Port=2  Side=Right
  wires:
  Bend/1 -> Simulink-PS Converter1/1
  Gain/1 -> Simulink-PS Converter/1
  Pitch Moment/1 -> Simulink-PS Converter2/1
  spin/1 -> Gain/1
  connections:
  External Force and Torque2/LConn2 -- Simulink-PS Converter1/RConn1 -- External Force and Torque1/LConn2
  B2/RConn1 -- External Force and Torque2/RConn1
  External Force and Torque2/LConn3 -- External Force and Torque1/LConn3 -- Simulink-PS Converter2/RConn1
  External Force and Torque2/LConn1 -- Simulink-PS Converter/RConn1 -- External Force and Torque1/LConn1
  B1/RConn1 -- External Force and Torque1/RConn1

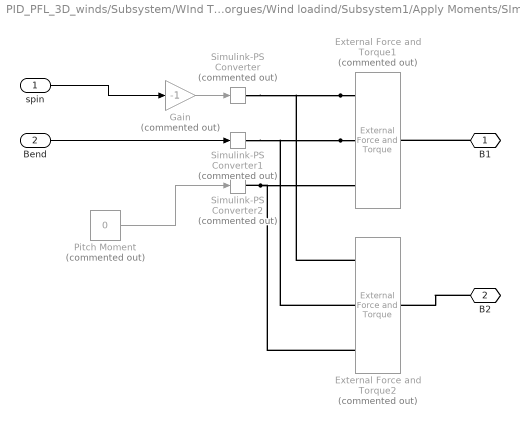
== system PID_PFL_3D_winds/Subsystem/WInd Torgues/Wind loadind/Subsystem1/Apply Moments/SImscape ==
  spin : Inport
  Bend : Inport  Port=2
  External Force and Torque1 : sm_lib/Forces and Torques/External Force and Torque  Commented=on  ForceResolutionFrame=AttachedFrame  EnableForceX=off  EnableForceY=off  EnableForceZ=off  EnableForce=off  TorqueResolutionFrame=AttachedFrame  EnableTorqueX=on  EnableTorqueY=on  EnableTorqueZ=on  EnableTorque=off
  External Force and Torque2 : sm_lib/Forces and Torques/External Force and Torque  Commented=on  ForceResolutionFrame=AttachedFrame  EnableForceX=off  EnableForceY=off  EnableForceZ=off  EnableForce=off  TorqueResolutionFrame=AttachedFrame  EnableTorqueX=on  EnableTorqueY=on  EnableTorqueZ=on  EnableTorque=off
  Gain : Gain  Commented=on  Gain=-1
  Pitch Moment : Constant  Commented=on  Value=0
  Simulink-PS Converter : nesl_utility/Simulink-PS Converter  Commented=on  PhysicalDomain=network_engine_domain  SubClassName=ps_input  LeftPortType=input  RightPortType=output  PseudoPeriodic=off  Frequencies=[]  NoiseDistribution=none  NoiseParameters=[]  Unit=1  AffineConversion=off  FilteringAndDerivatives=zero  SimscapeFilterOrder=1  InputFilterTimeConstant=0.005  UdotUserProvided=[]
  Simulink-PS Converter1 : nesl_utility/Simulink-PS Converter  Commented=on  PhysicalDomain=network_engine_domain  SubClassName=ps_input  LeftPortType=input  RightPortType=output  PseudoPeriodic=off  Frequencies=[]  NoiseDistribution=none  NoiseParameters=[]  Unit=1  AffineConversion=off  FilteringAndDerivatives=zero  SimscapeFilterOrder=1  InputFilterTimeConstant=0.005  UdotUserProvided=[]
  Simulink-PS Converter2 : nesl_utility/Simulink-PS Converter  Commented=on  PhysicalDomain=network_engine_domain  SubClassName=ps_input  LeftPortType=input  RightPortType=output  PseudoPeriodic=off  Frequencies=[]  NoiseDistribution=none  NoiseParameters=[]  Unit=1  AffineConversion=off  FilteringAndDerivatives=zero  SimscapeFilterOrder=1  InputFilterTimeConstant=0.005  UdotUserProvided=[]
  B1 : PMIOPort  Side=Right
  B2 : PMIOPort  Port=2  Side=Right
  wires:
  spin/1 -> Gain/1
  Pitch Moment/1 -> Simulink-PS Converter2/1
  Gain/1 -> Simulink-PS Converter/1
  Bend/1 -> Simulink-PS Converter1/1
  connections:
  B1/RConn1 -- External Force and Torque1/RConn1
  External Force and Torque1/LConn1 -- Simulink-PS Converter/RConn1 -- External Force and Torque2/LConn1
  Simulink-PS Converter2/RConn1 -- External Force and Torque1/LConn3 -- External Force and Torque2/LConn3
  B2/RConn1 -- External Force and Torque2/RConn1
  External Force and Torque1/LConn2 -- Simulink-PS Converter1/RConn1 -- External Force and Torque2/LConn2

== matlab function PID_PFL_3D_winds/PF Linearization Underactuated ==
  settings: updateMethod=DISCRETE
  data: tau_wristy output; tau_elbow output; u1 input; u2 input; u3 input; theta1x input; theta1y input; theta2 input; dtheta1x input; dtheta1y input; dtheta2 input
function [tau_wristy, tau_elbow] = compute_actuator_torques( ...
    u1, u2, u3, ...
    theta1x, theta1y, theta2, ...
    dtheta1x, dtheta1y, dtheta2)
% COMPUTE_ACTUATOR_TORQUES - self-contained, no structs used anywhere.
% Produces actuator torques for wrist-y (phi) and elbow (theta2).
%
% Call:
%  [tau_wristy, tau_elbow, term_gen] = compute_actuator_torques(u1,u2, ...
%       th1x, th1y, th2, dth1x, dth1y, dth2)

%% ---------------- Robot parameters (scalars only) -------------------
% Edit these values here if you want different robot parameters
m1  = 4.8;
m2  = 4.8;
l1  = 1.0;
l2  = 1.0;
lc1 = 0.5 * l1;
lc2 = 0.5 * l2;
I1  = (1/3) * m1 * l1^2;
I2  = (1/3) * m2 * l2^2;
fk1 = 0.3;
fk2 = 0.3;
g   = 9.81;
% optional torque limits:
% tau_phi_max = 5; tau_elbow_max = 10;

%% pack q/dq
q  = [theta1x; theta1y; theta2];
dq = [dtheta1x; dtheta1y; dtheta2];

%% compute dynamics (M, Cvec, G) using scalars (no struct)
[M, Cvec, G, B2, B3] = dynamics3d(q, dq, m1, m2, l1, l2, lc1, lc2, I1, I2, g);

%% generalized control input (u1 -> phi, u2 -> theta2)
u_gen = [u1; u2; u3];   % third entry corresponds to theta2 command

%% generalized torque target
term_gen = M * u_gen + Cvec + G;   % 3x1 generalized torque target

%% actuator torques (B2 = [0 0; 1 0; 0 1])
tau_wristy = term_gen(2);
tau_elbow  = term_gen(3);

% optional saturation (uncomment and set limits if desired)
% tau_wristy = max(-tau_phi_max, min(tau_phi_max, tau_wristy));
% tau_elbow  = max(-tau_elbow_max, min(tau_elbow_max, tau_elbow));

end


%% -------------------- dynamics helper (no struct) --------------------
function [M, Cvec, G, B2, B3] = dynamics3d(q, dq, m1, m2, l1, l2, lc1, lc2, I1, I2, g)
% Compute mass matrix M (3x3), coriolis/centrifugal vector Cvec (3x1),
% gravity G (3x1) and control maps B2/B3 for q = [th1; phi; th2].

th1 = q(1); phi = q(2); th2 = q(3);
dth1 = dq(1); dphi = dq(2); dth2 = dq(3);

% helpers
s1 = sin(th1); c1 = cos(th1);
s12 = sin(th1 + th2); c12 = cos(th1 + th2);

% Jv1 (link1 COM)
dr1_dth1 = lc1 * [ cos(th1)*cos(phi); cos(th1)*sin(phi); sin(th1) ];
dr1_dphi  = lc1 * [ -sin(th1)*sin(phi); sin(th1)*cos(phi); 0 ];
dr1_dth2 = [0;0;0];
Jv1 = [dr1_dth1, dr1_dphi, dr1_dth2];

% Jv2 (link2 COM)
A = l1*sin(th1) + lc2*sin(th1 + th2);
dA_dth1 = l1*cos(th1) + lc2*cos(th1 + th2);
dA_dth2 = lc2*cos(th1 + th2);

dr2_dth1 = [ dA_dth1 * cos(phi); dA_dth1 * sin(phi); (l1*sin(th1) + lc2*sin(th1+th2)) ];
dr2_dphi  = [ -A * sin(phi); A * cos(phi); 0 ];
dr2_dth2  = [ dA_dth2 * cos(phi); dA_dth2 * sin(phi); lc2 * sin(th1+th2) ];
Jv2 = [dr2_dth1, dr2_dphi, dr2_dth2];

% translational mass part
M_trans = m1 * (Jv1')*Jv1 + m2 * (Jv2')*Jv2;

% rotational inertia contributions (approx)
M_rot1 = I1 * [ 1,           0, 0;
                0, sin(th1)^2, 0;
                0,           0, 0 ];
M_rot2 = I2 * [ 1,                      0, 1;
                0, sin(th1+th2)^2,      0;
                1,                      0, 1 ];

M = M_trans + M_rot1 + M_rot2;

% gravity vector
G1 = g*( m1*lc1*sin(th1) + m2*( l1*sin(th1) + lc2*sin(th1+th2) ) );
G2 = 0;
G3 = g*( m2*lc2*sin(th1+th2) );
G  = [G1; G2; G3];

% compute Coriolis/centrifugal vector Cvec (numeric Christoffel)
n = 3;
Cvec = zeros(n,1);
dM = zeros(n,n,n);
eps_der = 1e-7;  % small step for numeric derivative
for k = 1:n
    dqk = zeros(n,1); dqk(k) = eps_der;
    q_plus = q + dqk;
    Mplus = computeM_numeric(q_plus, m1, m2, l1, l2, lc1, lc2, I1, I2);
    dM(:,:,k) = (Mplus - M) / eps_der;  % dM(i,j,k) = d/dq_k M(i,j)
end
for k = 1:n
    s = 0;
    for i = 1:n
        for j = 1:n
            Gamma_kij = 0.5 * ( dM(k,j,i) + dM(k,i,j) - dM(i,j,k) );
            s = s + Gamma_kij * dq(i) * dq(j);
        end
    end
    Cvec(k) = s;
end

% control maps (actuators: tau_phi, tau_elbow)
B2 = [0 0; 1 0; 0 1];
B3 = eye(3);

end


%% --------------- computeM_numeric (no struct) -----------------------
function Mloc = computeM_numeric(q, m1, m2, l1, l2, lc1, lc2, I1, I2)
% Compute mass matrix given q and scalar params.

th1 = q(1); phi = q(2); th2 = q(3);

% Jv1
dr1_dth1 = lc1 * [ cos(th1)*cos(phi); cos(th1)*sin(phi); sin(th1) ];
dr1_dphi  = lc1 * [ -sin(th1)*sin(phi); sin(th1)*cos(phi); 0 ];
dr1_dth2 = [0;0;0];
Jv1 = [dr1_dth1, dr1_dphi, dr1_dth2];

% Jv2
A = l1*sin(th1) + lc2*sin(th1+th2);
dA_dth1 = l1*cos(th1) + lc2*cos(th1+th2);
dA_dth2 = lc2*cos(th1+th2);
dr2_dth1 = [ dA_dth1 * cos(phi); dA_dth1 * sin(phi); (l1*sin(th1) + lc2*sin(th1+th2)) ];
dr2_dphi  = [ -A * sin(phi); A * cos(phi); 0 ];
dr2_dth2  = [ dA_dth2 * cos(phi); dA_dth2 * sin(phi); lc2 * sin(th1+th2) ];
Jv2 = [dr2_dth1, dr2_dphi, dr2_dth2];

M_trans = m1 * (Jv1')*Jv1 + m2 * (Jv2')*Jv2;

M_rot1 = I1 * [ 1,           0, 0;
                0, sin(th1)^2, 0;
                0,           0, 0 ];
M_rot2 = I2 * [ 1,                      0, 1;
                0, sin(th1+th2)^2,      0;
                1,                      0, 1 ];

Mloc = M_trans + M_rot1 + M_rot2;
end

== matlab function PID_PFL_3D_winds/Subsystem/WInd Torgues/Unsteady Wind Velocities ==
  settings: updateMethod=DISCRETE
  data: U_R1 output; U_R2 output; windSpeed input
function [U_R1, U_R2] = fcn(windSpeed)
    alpha = 0.244;
    sigma = 1;
    theta1 = 1.23;
    theta2 = -1.24;

    if windSpeed == 0
      u_p = 0;  v_p = 0;  w_p = 0;
    else
      u_p = sigma*randn(1,1);
      v_p = sigma*randn(1,1);
      w_p = sigma*randn(1,1);
    end
 % Calculate components of the relative velocity
    U_x = windSpeed + u_p;
    U_y = v_p;
    U_z = w_p;

  % Apply transformation matrix 1
    % first link
    U_xp = U_x*cos(theta1)*cos(alpha) - U_y*sin(alpha) + U_z*sin(theta1)*cos(alpha);
    U_yp = U_x*cos(theta1)*sin(alpha) + U_y*cos(alpha) + U_z*sin(theta1)*sin(alpha);
    U_zp = -U_x*sin(theta1)             + U_z*cos(theta1);
    U_R1  = sqrt(U_xp.^2 + U_yp.^2 + U_zp.^2);

      % Apply transformation matrix 2
    % second link 
    U_xp2 = U_x*cos(theta2)*cos(alpha) - U_y*sin(alpha) + U_z*sin(theta2)*cos(alpha);
    U_yp2 = U_x*cos(theta2)*sin(alpha) + U_y*cos(alpha) + U_z*sin(theta2)*sin(alpha);
    U_zp2 = -U_x*sin(theta2)             + U_z*cos(theta2);
    U_R2  = sqrt(U_xp2.^2 + U_yp2.^2 + U_zp2.^2);
end

== matlab function PID_PFL_3D_winds/Subsystem/MATLAB Function ==
  data: x2 output; theta1x input; y2 output; theta2 input; theta1y input; z2 output
function [x2, y2, z2] = fcn(theta1x, theta2, theta1y)
%FCN 3D forward kinematics for a 2-link pendulum where the first joint
% provides an out-of-plane yaw (theta1z).
%
% Inputs:
%   theta1  - first link polar angle (rad). (your theta1x)
%   theta2  - second link relative angle (rad)
%   theta1z - yaw/azimuth of link-1 about vertical axis (rad)
%
% Outputs:
%   x2, y2, z2 - 3D end-effector coordinates (meters)
%
% Note: link lengths are set to l1 = l2 = 1 (same as your original function).
%       If you need different link lengths, change l1 and l2 or pass them in.

%#codegen

% link lengths (change if needed)
l1 = 1;
l2 = 1;

% --- plan view (sagittal-plane) coordinates before yaw rotation ---
% forward direction (along X before yaw) in sagittal plane:
x_planar = l1 .* sin(theta1x) + l2 .* sin(theta1x + theta2);

% vertical coordinate (Z, "down" positive if following your previous sign convention)
z2 = - ( l1 .* cos(theta1x) + l2 .* cos(theta1x + theta2) );

% yaw (rotation about global Z) rotates the planar forward coordinate into X,Y
% assume the sagittal plane initially lies along the global X axis (y=0).
x2 = x_planar .* cos(theta1y);
y2 = x_planar .* sin(theta1y);

end
